simulink model "DIYcontroller"  (R2021a)
settings: Solver=FixedStepAuto  StartTime=0.0  StopTime=10.0  FixedStep=0.001  RelTol=1e-3
values from neighbouring files (symbols this model uses):
  Vx = 15    [controller_setup.m]
libraries: robotlib x22, simulink x1
settings Model: Creator=chnwa  LastModifiedBy=chnwa
settings OptimizationCC: EnhancedBackFolding=on  PassReuseOutputArgsAs=Individual arguments  ZeroExternalMemoryAtStartup=off  ZeroInternalMemoryAtStartup=off  MaxStackSize=64  OptimizeBlockOrder=speed  DifferentSizesBufferReuse=on  OptimizationCustomize=off  EfficientTunableParamExpr=on
settings DebuggingCC: ParameterTunabilityLossMsg=error
settings HardwareCC: ProdBitPerPointer=32  ProdBitPerSizeT=32  ProdBitPerPtrDiffT=32  ProdLargestAtomicFloat=None  ProdIntDivRoundTo=Undefined  ProdEndianess=Unspecified  ProdWordSize=32  ProdHWDeviceType=Generic->Unspecified (assume 32-bit Generic)
settings SFSimCC: MATLABDynamicMemAlloc=off
settings RTWCC: SystemTargetFile=ert.tlc  HardwareBoard=Robot Operating System (ROS)  TLCOptions="-aInlineSetEventsForThisBaseRateFcn=TLC_FALSE -aSuppressMultiTaskScheduler=TLC_FALSE  -aRateBasedStepFcn=0"  TemplateMakefile=ert_default_tmf  Toolchain=Catkin  TargetLang=C++
settings CodeAppCC: ForceParamTrailComments=on  IgnoreCustomStorageClasses=off  OperatorAnnotations=on  SimulinkDataObjDesc=on  SFDataObjDesc=on  InsertBlockDesc=on
settings ERTTargetCC: SupportVariableSizeSignals=on

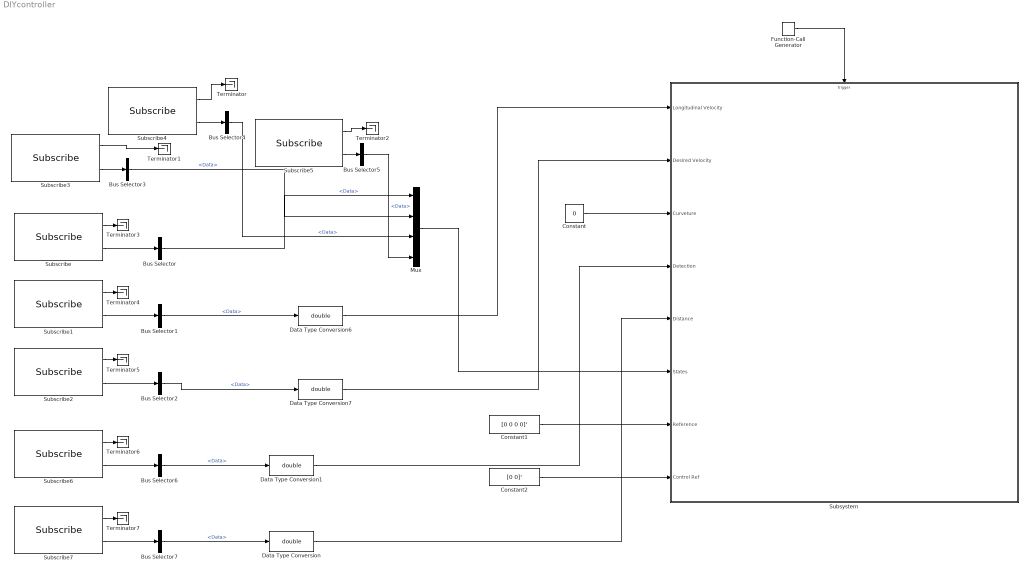
== system DIYcontroller ==
  Bus Selector{,1..7} (8 alike) : BusSelector  OutputSignals=Data
  Constant : Constant  Value=0
  Constant1 : Constant  Value=[0 0 0 0]'
  Constant2 : Constant  Value=[0 0]'
  Data Type Conversion{,1,6..7} (4 alike) : DataTypeConversion  OutDataTypeStr=double
  Function-Call Generator : simulink/Ports & Subsystems/Function-Call Generator  sample_time=0.05  numberOfIterations=1  DisallowWideOutput=off
  Mux : Mux
  Subscribe : robotlib/Subscribe  topicSource=Specify your own  topic=/states1  messageType=std_msgs/Float64  SampleTime=-1  legacyBusStruct=off  messageQueueLength=1
  Subscribe1 : robotlib/Subscribe  topicSource=Specify your own  topic=/Vx  messageType=std_msgs/Float64  SampleTime=-1  legacyBusStruct=off  messageQueueLength=1
  Subscribe2 : robotlib/Subscribe  topicSource=Specify your own  topic=/Vset  messageType=std_msgs/Float64  SampleTime=-1  legacyBusStruct=off  messageQueueLength=1
  Subscribe3 : robotlib/Subscribe  topicSource=Specify your own  topic=/states2  messageType=std_msgs/Float64  SampleTime=-1  legacyBusStruct=off  messageQueueLength=1
  Subscribe4 : robotlib/Subscribe  topicSource=Specify your own  topic=/states3  messageType=std_msgs/Float64  SampleTime=-1  legacyBusStruct=off  messageQueueLength=1
  Subscribe5 : robotlib/Subscribe  topicSource=Specify your own  topic=/states4  messageType=std_msgs/Float64  SampleTime=-1  legacyBusStruct=off  messageQueueLength=1
  Subscribe6 : robotlib/Subscribe  topicSource=Specify your own  topic=/Detection  messageType=std_msgs/Float64  SampleTime=-1  legacyBusStruct=off  messageQueueLength=1
  Subscribe7 : robotlib/Subscribe  topicSource=Specify your own  topic=/Distance  messageType=std_msgs/Float64  SampleTime=-1  legacyBusStruct=off  messageQueueLength=1
  Subsystem : Subsystem
  Terminator{,1..7} (8 alike) : Terminator
  wires:
  Subscribe1/1 -> Terminator4/1
  Subscribe4/1 -> Terminator/1
  Subscribe6/2 -> Bus Selector6/1
  Bus Selector3/1 -> Mux/2  "<Data>"
  Subscribe/1 -> Terminator3/1
  Subscribe/2 -> Bus Selector/1
  Subscribe4/2 -> Bus Selector4/1
  Subscribe2/2 -> Bus Selector2/1
  Subscribe3/1 -> Terminator1/1
  Bus Selector5/1 -> Mux/4  "<Data>"
  Subscribe2/1 -> Terminator5/1
  Bus Selector4/1 -> Mux/3  "<Data>"
  Subscribe1/2 -> Bus Selector1/1
  Subscribe6/1 -> Terminator6/1
  Subscribe3/2 -> Bus Selector3/1
  Bus Selector/1 -> Mux/1  "<Data>"
  Subscribe5/2 -> Bus Selector5/1
  Subscribe5/1 -> Terminator2/1
  Bus Selector1/1 -> Data Type Conversion6/1  "<Data>"
  Bus Selector2/1 -> Data Type Conversion7/1  "<Data>"
  Function-Call Generator/1 -> Subsystem/Trigger
  Subscribe7/1 -> Terminator7/1
  Subscribe7/2 -> Bus Selector7/1
  Bus Selector6/1 -> Data Type Conversion1/1  "<Data>"
  Bus Selector7/1 -> Data Type Conversion/1  "<Data>"
  Data Type Conversion/1 -> Subsystem/5(Distance)
  Data Type Conversion1/1 -> Subsystem/4(Detection)
  Data Type Conversion6/1 -> Subsystem/1(Longitudinal Velocity)
  Data Type Conversion7/1 -> Subsystem/2(Desired Velocity)
  Constant/1 -> Subsystem/3(Curveture)
  Mux/1 -> Subsystem/6(States)
  Constant1/1 -> Subsystem/7(Reference)
  Constant2/1 -> Subsystem/8(Control Ref)

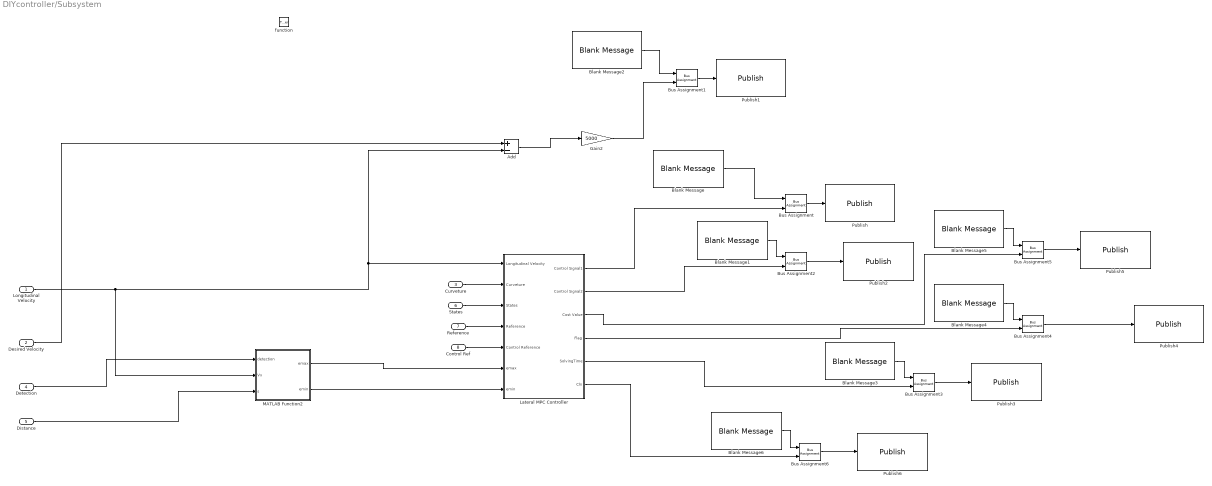
== system DIYcontroller/Subsystem ==
  Longitudinal Velocity : Inport
  Desired Velocity : Inport  Port=2
  Curveture : Inport  Port=3
  Detection : Inport  Port=4
  Distance : Inport  Port=5
  States : Inport  Port=6
  Reference : Inport  Port=7
  Control Ref : Inport  Port=8
  function : TriggerPort  TriggerType=function-call  VariantControl=(inherit)
  Add : Sum  Inputs=+-
  Blank Message{,1..6} (7 alike) : robotlib/Blank Message  messageClass=Message  entityType=std_msgs/Float64  messageType=std_msgs/Float64  SampleTime=inf  legacyBusStruct=off
  Bus Assignment{,1..6} (7 alike) : BusAssignment  AssignedSignals=Data
  Gain2 : Gain  Gain=5000
  Lateral MPC Controller : Subsystem
  MATLAB Function2 : MATLAB Function  TreatAsAtomicUnit=on
  Publish : robotlib/Publish  topicSource=Specify your own  topic=/ControlInput1  messageType=std_msgs/Float64  legacyBusStruct=off  messageQueueLength=1
  Publish1 : robotlib/Publish  topicSource=Specify your own  topic=/Fxnet  messageType=std_msgs/Float64  legacyBusStruct=off  messageQueueLength=1
  Publish2 : robotlib/Publish  topicSource=Specify your own  topic=/ControlInput2  messageType=std_msgs/Float64  legacyBusStruct=off  messageQueueLength=1
  Publish3 : robotlib/Publish  topicSource=Specify your own  topic=/Time  messageType=std_msgs/Float64  legacyBusStruct=off  messageQueueLength=1
  Publish4 : robotlib/Publish  topicSource=Specify your own  topic=/Flag  messageType=std_msgs/Float64  legacyBusStruct=off  messageQueueLength=1
  Publish5 : robotlib/Publish  topicSource=Specify your own  topic=/CostValue  messageType=std_msgs/Float64  legacyBusStruct=off  messageQueueLength=1
  Publish6 : robotlib/Publish  topicSource=Specify your own  topic=/Chi  messageType=std_msgs/Float64  legacyBusStruct=off  messageQueueLength=1
  wires:
  Bus Assignment/1 -> Publish/1
  Longitudinal Velocity/1 -> MATLAB Function2/2(Vx), Add/2, Lateral MPC Controller/1(Longitudinal Velocity)
  Curveture/1 -> Lateral MPC Controller/2(Curveture)
  Blank Message1/1 -> Bus Assignment2/1
  Bus Assignment2/1 -> Publish2/1
  Blank Message2/1 -> Bus Assignment1/1
  Blank Message/1 -> Bus Assignment/1
  Add/1 -> Gain2/1
  Bus Assignment1/1 -> Publish1/1
  Gain2/1 -> Bus Assignment1/2
  Desired Velocity/1 -> Add/1
  Blank Message3/1 -> Bus Assignment3/1
  Bus Assignment3/1 -> Publish3/1
  Lateral MPC Controller/5(SolvingTime) -> Bus Assignment3/2
  Blank Message4/1 -> Bus Assignment4/1
  Bus Assignment4/1 -> Publish4/1
  Lateral MPC Controller/4(Flag) -> Bus Assignment4/2
  Blank Message5/1 -> Bus Assignment5/1
  Bus Assignment5/1 -> Publish5/1
  Detection/1 -> MATLAB Function2/1(detection)
  Distance/1 -> MATLAB Function2/3(s)
  MATLAB Function2/1(emax) -> Lateral MPC Controller/6(emax)
  MATLAB Function2/2(emin) -> Lateral MPC Controller/7(emin)
  Lateral MPC Controller/2(Control Signal2) -> Bus Assignment2/2
  Lateral MPC Controller/1(Control Signal1) -> Bus Assignment/2
  Lateral MPC Controller/3(Cost Value) -> Bus Assignment5/2
  States/1 -> Lateral MPC Controller/3(States)
  Reference/1 -> Lateral MPC Controller/4(Reference)
  Control Ref/1 -> Lateral MPC Controller/5(Control Reference)
  Lateral MPC Controller/6(Chi) -> Bus Assignment6/2
  Bus Assignment6/1 -> Publish6/1
  Blank Message6/1 -> Bus Assignment6/1

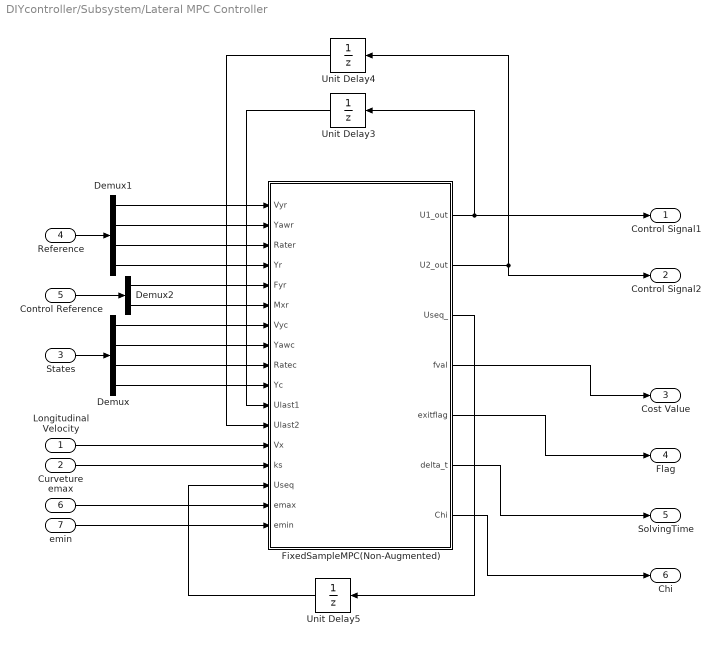
== system DIYcontroller/Subsystem/Lateral MPC Controller ==
  Longitudinal Velocity : Inport
  Curveture : Inport  Port=2
  States : Inport  Port=3
  Reference : Inport  Port=4
  Control Reference : Inport  Port=5
  emax : Inport  Port=6
  emin : Inport  Port=7
  Demux : Demux
  Demux1 : Demux
  Demux2 : Demux  Outputs=2
  FixedSampleMPC(Non-Augmented) : MATLAB Function  TreatAsAtomicUnit=on
  Unit Delay3 : UnitDelay  SampleTime=-1  HasFrameUpgradeWarning=on
  Unit Delay4 : UnitDelay  SampleTime=-1  HasFrameUpgradeWarning=on
  Unit Delay5 : UnitDelay  InitialCondition=zeros(61,2)  SampleTime=-1  HasFrameUpgradeWarning=on
  Control Signal1 : Outport
  Control Signal2 : Outport  Port=2
  Cost Value : Outport  Port=3
  Flag : Outport  Port=4
  SolvingTime : Outport  Port=5
  Chi : Outport  Port=6
  wires:
  FixedSampleMPC(Non-Augmented)/5(exitflag) -> Flag/1
  FixedSampleMPC(Non-Augmented)/2(U2_out) -> Control Signal2/1, Unit Delay4/1
  Unit Delay4/1 -> FixedSampleMPC(Non-Augmented)/12(Ulast2)
  Longitudinal Velocity/1 -> FixedSampleMPC(Non-Augmented)/13(Vx)
  Demux/3 -> FixedSampleMPC(Non-Augmented)/9(Ratec)
  FixedSampleMPC(Non-Augmented)/3(Useq_) -> Unit Delay5/1
  Demux/1 -> FixedSampleMPC(Non-Augmented)/7(Vyc)
  FixedSampleMPC(Non-Augmented)/4(fval) -> Cost Value/1
  Curveture/1 -> FixedSampleMPC(Non-Augmented)/14(ks)
  emax/1 -> FixedSampleMPC(Non-Augmented)/16(emax)
  Demux/2 -> FixedSampleMPC(Non-Augmented)/8(Yawc)
  Demux/4 -> FixedSampleMPC(Non-Augmented)/10(Yc)
  FixedSampleMPC(Non-Augmented)/1(U1_out) -> Unit Delay3/1, Control Signal1/1
  Unit Delay5/1 -> FixedSampleMPC(Non-Augmented)/15(Useq)
  Unit Delay3/1 -> FixedSampleMPC(Non-Augmented)/11(Ulast1)
  FixedSampleMPC(Non-Augmented)/6(delta_t) -> SolvingTime/1
  emin/1 -> FixedSampleMPC(Non-Augmented)/17(emin)
  States/1 -> Demux/1
  Reference/1 -> Demux1/1
  Demux1/1 -> FixedSampleMPC(Non-Augmented)/1(Vyr)
  Demux1/2 -> FixedSampleMPC(Non-Augmented)/2(Yawr)
  Demux1/3 -> FixedSampleMPC(Non-Augmented)/3(Rater)
  Demux1/4 -> FixedSampleMPC(Non-Augmented)/4(Yr)
  Control Reference/1 -> Demux2/1
  Demux2/1 -> FixedSampleMPC(Non-Augmented)/5(Fyr)
  Demux2/2 -> FixedSampleMPC(Non-Augmented)/6(Mxr)
  FixedSampleMPC(Non-Augmented)/7(Chi) -> Chi/1

== matlab function DIYcontroller/Subsystem/MATLAB Function2 ==
  data: detection input; Vx input size=1; s input; emax output; emin output
function [emax,emin] = fcn(detection,Vx,s)
PredictionHorizon=60;
Ts=0.05;
k = round(s/Vx/Ts);
if k>PredictionHorizon
    k =PredictionHorizon;
elseif k<20
    k=20;
end

if detection == 1
    emin = -10*ones(PredictionHorizon,1);
    emax=   10*ones(PredictionHorizon,1);
    k1=k-round(3/Vx/Ts);
    k2=k+round(3/Vx/Ts);
    if k1<1
        k1=1;
    end
    if k2>PredictionHorizon
        k2=PredictionHorizon;
    end
    emin(k1:k2)=4;
    emax(k1:k2)=6;
else
    emin=-10*ones(PredictionHorizon,1);
    emax=10*ones(PredictionHorizon,1);
end

== matlab function DIYcontroller/Subsystem/Lateral MPC Controller/FixedSampleMPC(Non-Augmented) ==
  data: Vyr input; U1_out output; Yawr input; Rater input; Yr input; Fyr input; Mxr input; Vyc input; Yawc input; Ratec input; Yc input; Ulast1 input; Ulast2 input; Vx input; ks input; Useq input; U2_out output; Useq_ output; fval output; exitflag output; delta_t output; emax input; emin input; Chi output
function [U1_out,U2_out,Useq_,fval,exitflag,delta_t,Chi] = fcn(Vyr,Yawr,Rater,Yr, Fyr,Mxr,Vyc,Yawc,Ratec,Yc,Ulast1,Ulast2,Vx,ks,Useq,emax,emin)
%Vyr lateral velocity, Yawr yaw angle, Rater yaw rate, Yr lateral position
%Fyr lateral force in front tyre,Mxr moment generated by longitudinal force
%'r'means reference ||  'c'means current
    if Vx<0.1
        Vx=0.001;%make sure many expressions' denominator isn't 0
    end
    lr=1.67;
    threshold=0.1022; %largest rear slip angle in linear region
    miu=0.7;
    rmax=9.81*miu/Vx;
%% Initilization    
    tstart=tic;%timing on
    
    Nx=4;%number of state
    Nu=2;%number of control
    Np=60;%prediction horizon
    Nc=1;%control horizon

    %reference
    r=zeros(Nx,1);%state reference
    r(1)=Vyr;
    r(2)=Yawr;
    r(3)=Rater;
    r(4)=Yr;    
    ur1=Fyr;
    ur2=Mxr;%control reference
    
    %states
    x=zeros(Nx,1);%state reference
    x(1)=Vyc;
    x(2)=Yawc;
    x(3)=Ratec;
    x(4)=Yc;   
    
    %control
    u=zeros(Nu,1);%state reference
    u(1)=Ulast1;
    u(2)=Ulast2;
    
    %get augmented states
    kesi=zeros(Nx+Nu,1);%[X;U]
    kesi(1)=x(1)-r(1);
    kesi(2)=x(2)-r(2);
    kesi(3)=x(3)-r(3);
    kesi(4)=x(4)-r(4);
    kesi(5)=u(1)-ur1;
    kesi(6)=u(2)-ur2;
    
    Ts=0.05;%sample time
    
%% Modellng->Discretization->prediction->quadratic programming
    %Modelling&Linearization&Discretization
    steps=Np+1;
    A = zeros(Nx+Nu,Nx+Nu,steps);
    B = zeros(Nx+Nu,Nu,steps);
    Dc = zeros(Nx+Nu,1,steps);
    C=[1 0 0 0 0 0;0 1 0 0 0 0;0 0 1 0 0 0;0 0 0 1 0 0];
    
    for ct = 1:steps
        if ct>length(Useq)
            uk = Useq(Np,:);
        else
            uk = Useq(ct,:);
        end
        uk=uk';
        [Ad, Bd, DK, delta_x] = GetDynamics(Vx,ks,x,uk,Ts);
        A(:,:,ct)=[Ad,Bd;zeros(Nu,Nx),eye(Nu)];        
        B(:,:,ct)=[Bd;eye(Nu)];
        Dc(:,:,ct)=[DK;0;0];
        x=x+delta_x;    
    end
    %construct important matrix
    %Y=PHI*kesi+THETA*delta_U+OMEGA*D
    coder.varsize('PHI',[Np*Nx,Nx+Nu]);
    coder.varsize('THETA',[Np*Nx,Nc*Nu]);
    coder.varsize('D',[Np*(Nx+Nu),1]);
    coder.varsize('DD',[Np*Nx,1]);
    PHI=[];
    THETA=[];
    D=[];
    DD=[];
    product=eye(6);
    for j=1:Np
        product=A(:,:,j)*product;
        PHI=[PHI;C*product];
        D=[D;Dc(:,:,j)];
    end
    for k=1:Nc
        product1=eye(6);
        for j=1:Np
            THETA=[THETA;C*product1*B(:,:,k)];
            product1=A(:,:,j+1)*product1;
        end
    end
    coder.varsize('OMEGA',[Nx*Np,(Nx+Nu)*Np]);
    OMEGA=zeros(Nx*Np,(Nx+Nu)*Np);
    for i=1:Np
        product2=A(:,:,i+1);
        for j=i:Np-1
            if i==j
                OMEGA(4*i-3:4*i,6*i-5:6*i)=C*eye(6);
            end
            OMEGA(4*j+1:4*j+4,6*j+1:6*j+6)=C*product2;
            product2=A(:,:,j+2)*product2;
        end
    end
    DD=OMEGA*D;        
    Sigma=zeros(Np,Nc);
    for p=1:Np%define a lower triangular matrix
        for q=1:1:Nc
            if q<=p 
                Sigma(p,q)=1;
            else 
                Sigma(p,q)=0;
            end
        end 
    end 
    UT=kron(ones(Np,1),[u(1);u(2)]);
    Sigma=kron(Sigma,eye(Nu));
    error=PHI*kesi;
    Q=kron(eye(Np,Np),diag([0 0 100 4]));    
    R=kron(eye(Np,Np),diag([0 4e-5]));    
    P=diag([3e-5 8e-5]);
    rou1=3e3;    
    rou2=5e4;
    H=2*[THETA'*Q*THETA+Sigma'*R*Sigma+P zeros(2,2);0 0 rou1 0;0 0 0 rou2];%是否要乘2？要
    f=[2*(error'*Q*THETA+(OMEGA*D)'*Q*THETA+UT'*R*Sigma),0,0];%是否要转置？好像无所谓
   %% constraints
    if abs(x(2))<=rmax
        Chi1=1;
    elseif abs(x(2))>rmax&&abs(x(2))<=(1+0.1)*rmax
        Chi1=1-(abs(x(2)-rmax))/(0.1*rmax);
    else
        Chi1=0;
    end
    alphar=(x(1)-lr*x(2))/Vx; %alphar is the slip angle of rear tyre
    if abs(alphar)<=threshold
        Chi2=1;
    elseif abs(alphar)>threshold&&abs(alphar)<=(1+0.1)*threshold
        Chi2=1-(abs(alphar)-threshold)/(0.1*threshold);
    else
        Chi2=0;
    end
    Chi=min(Chi1,Chi2);%Chi adjusts the max allowable moments generated by longitudinal forces, lower it as it moves out of the parrallelogram
    %inequation
    A_t=zeros(Nc,Nc);
    for p=1:1:Nc%define a lower triangular matrix
        for q=1:1:Nc
            if q<=p 
                A_t(p,q)=1;
            else 
                A_t(p,q)=0;
            end
        end 
    end 
    A_I=kron(A_t,eye(Nu)); 
    Ut=kron(ones(Nc,1),[Ulast1;Ulast2]);%control in last control step
    umin=[-1e4; -1e3*Chi];
    umax=[1e4; 1e3*Chi];
    Umin=kron(ones(Nc,1),umin);
    Umax=kron(ones(Nc,1),umax);
    coder.varsize('A_cons',[Np*6+4,4]);
    coder.varsize('b_cons',[Np*6+4,1]);
    A_cons=[A_I zeros(Nu*Nc,2);-A_I zeros(Nu*Nc,2)];
    b_cons=[Umax-Ut;-Umin+Ut];
    %add handling envelop constriants & environment envolop
    gamas=[1 -lr 0 0;-1 lr 0 0;0 1 0 0;0 -1 0 0];
    gamae=[0 0 0 1;0 0 0 -1];
    Gs=[Vx*threshold;Vx*threshold;rmax;rmax];
    for i=1:Np
        A_cons=[A_cons;[gamas*THETA(4*i-3:4*i,:) -ones(4,1) zeros(4,1)];[gamae*THETA(4*i-3:4*i,:) zeros(2,1) -ones(2,1)]];
        b_cons=[b_cons;[Gs-gamas*(PHI(4*i-3:4*i,:)*kesi-DD(4*i-3:4*i,:))];[emax(i);-emin(i)]-gamae*(PHI(4*i-3:4*i,:)*kesi-DD(4*i-3:4*i,:))];
    end
    
    %upper and lower boundary
    delta_umin=[-1e4;-1e3];
    delta_umax=[1e4;1e3];
    M1=10; %related to slack variable
    M2=10; %related to slack variable
    delta_Umin=kron(ones(Nc,1),delta_umin);
    delta_Umax=kron(ones(Nc,1),delta_umax);
    lb=[delta_Umin;0;0];
    ub=[delta_Umax;M1;M2];  
   %% solve quadratic programming
    opts = optimoptions('quadprog','Algorithm','active-set');
    x_start=zeros(Nu*Nc+2,1);%+2 corresponds to slack variables
    [X,fval,exitflag]=quadprog(H,f',A_cons,b_cons,[],[],lb,ub,x_start,opts);
    
   %% calculate control signal
    U1=kesi(5)+X(1);%The output error at the previous time plus the optimization result to get the error at this time
    U2=kesi(6)+X(2);%The output error at the previous time plus the optimization result to get the error at this time
    U1_out=U1+ur1;%Error plus reference value to get final output value    
    U2_out=U2+ur2;
    Useq_=repmat([U1,U2],Np+1,1); %adaptive MPC block's method
%     Useq_=[[U1,U2];repmat(zeros(1,2),Np,1)]; %this may make more sense
    delta_t=toc(tstart);%timing off
end

function [A, B, DK, delta_x] = GetDynamics(Vx,ks,x,u,Ts)
%Plant Model parameters
m = 2272;   %mass
Iz = 4600;  %rotational inertia
lf = 1.11;  % distance from front axle to the mass center
lr = 1.67;  % distance from rear axle to the mass center
C_a = 1.822e5; % rear cornering stiffness 

%Enviroment parameters
miu = 0.7; %frction cooeficient 0.7 for dry road and 0.4 for wet
g = 9.81; % gravity

Fz = m*g*lf/(lf+lr); % the load that beared by the rear tire

%calculate alpha
Vy = x(1); %lateral velocity
r = x(2);  %yaw rate
alphar_ = Vy/Vx-lr*r/Vx;   %calculate linearzing point

%tire model
threshold = atan(3*miu*Fz/C_a);     % threshold for the tire linear region
if abs(alphar_)<threshold
    %the rear lateral force value (f(x0)) at the linearzing point
    Fyr_ = -C_a*tan(alphar_)+C_a^2/(3*miu*Fz)*abs(tan(alphar_))*tan(alphar_)-C_a^3/(27*miu^2*Fz^2)*tan(alphar_)^3;
    
    %the slope of linearized model (f‘(x0))
    if alphar_>= 0
        Cr_ = -C_a*sec(alphar_)^2+C_a^2/(3*miu*Fz)*(2*sec(alphar_)^2*tan(alphar_))-C_a^3/(27*miu^2*Fz^2)*(3*tan(alphar_)^2*sec(alphar_)^2);
    else
        Cr_ = -C_a*sec(alphar_)^2-C_a^2/(3*miu*Fz)*(2*sec(alphar_)^2*tan(alphar_))-C_a^3/(27*miu^2*Fz^2)*(3*tan(alphar_)^2*sec(alphar_)^2);
    end
else
    
    %the saturation region of tire model
    Fyr_ = -miu*Fz*sign(alphar_);
    Cr_ = 0;
end

%Continuous-time model
Ac = [Cr_/(m*Vx) -lr*Cr_/(m*Vx)-Vx 0 0;
    -lr*Cr_/(Iz*Vx) lr^2*Cr_/(Iz*Vx) 0 0;
    0 1 0 0;
    1 0 Vx 0];
Bc = [1/m 0;
    lf/Iz 1/Iz;
    0 0;
    0 0];
dcc = [(Fyr_-Cr_*alphar_)/m;
    -lr*(Fyr_-Cr_*alphar_)/Iz;
    -Vx*ks;
    0];

G=[Ac Bc dcc;zeros(3,7)];
M=expm(G*Ts);
A=M(1:4,1:4);
B=M(1:4,5:6);
DK=M(1:4,7);
delta_x=A*x+B*u+DK-x;
end
